simulink model "schema_pendolo"  (R2015a)
settings: Solver=ode45  StartTime=t(1)  StopTime=t(end)  MaxStep=5e-2  RelTol=1e-5
values from neighbouring files (symbols this model uses):
  g = 9.81    [InitPendolo.m]
  l = 1    [InitPendolo.m]
  m = 2    [InitPendolo.m]
  theta0 = 0.05*pi    (= 0.157079632679)    [InitPendolo.m]
  w0 = 0    [InitPendolo.m]
settings Model: Creator=Adriano  LastModifiedBy=Adriano

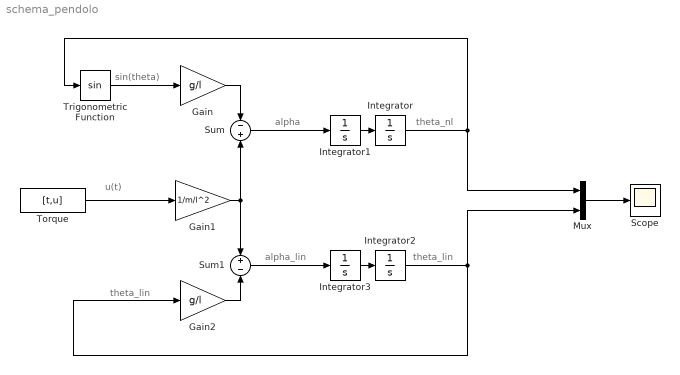
== system schema_pendolo ==
  note: theta_lin
  note: sin(theta)
  note: alpha_lin
  note: alpha
  note: theta_lin
  note: theta_nl
  note: u(t)
  Gain : Gain  Gain=g/l
  Gain1 : Gain  Gain=1/m/l^2
  Gain2 : Gain  Gain=g/l
  Integrator : Integrator  InitialCondition=theta0
  Integrator1 : Integrator  InitialCondition=w0
  Integrator2 : Integrator  InitialCondition=theta0
  Integrator3 : Integrator  InitialCondition=w0
  Mux : Mux  Inputs=2
  Scope : Scope
      settings: SaveName=simx
  Sum : Sum  Inputs=-|+
  Sum1 : Sum  Inputs=+|-
  Torque : FromWorkspace  VariableName=[t,u]  SampleTime=0
  Trigonometric Function : Trigonometry
  wires:
  Trigonometric Function/1 -> Gain/1
  Gain/1 -> Sum/1
  Integrator1/1 -> Integrator/1
  Sum/1 -> Integrator1/1
  Integrator/1 -> Mux/1, Trigonometric Function/1
  Gain1/1 -> Sum/2, Sum1/1
  Mux/1 -> Scope/1
  Torque/1 -> Gain1/1
  Integrator2/1 -> Gain2/1, Mux/2
  Gain2/1 -> Sum1/2
  Integrator3/1 -> Integrator2/1
  Sum1/1 -> Integrator3/1
